simulink subsystem "Actuatormodel_R2019B"  (R2019b)
settings: Solver=VariableStepAuto  StartTime=0.0  StopTime=10.0  RelTol=1e-3
undefined symbols (not defined in the file): act, DiscIntNeverNeededParam
settings Model: Creator=dylaneijkelhof  LastModifiedBy=dylaneijkelhof

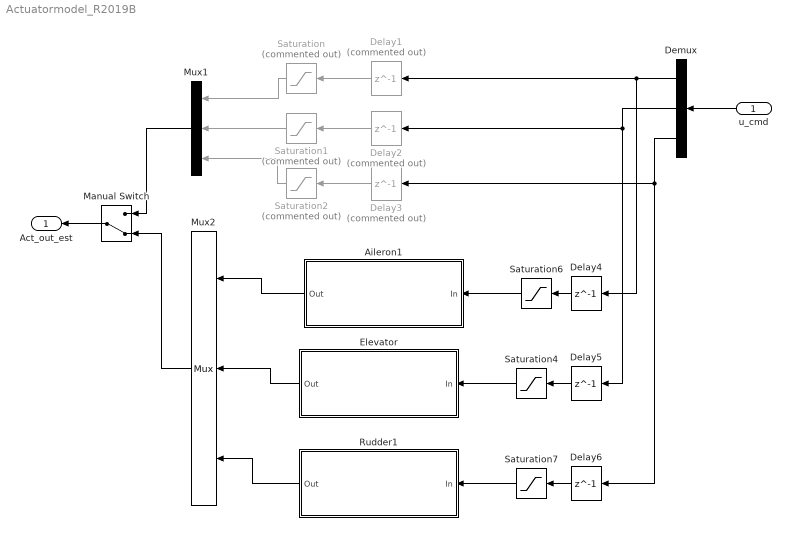
== system Actuatormodel_R2019B ==
  u_cmd : Inport
  Aileron1 : Subsystem  mask(Rate and Position Limited Servo){freq=act.aileron.w0/(2*pi), RL=act.aileron.rl, POS_hi=act.aileron.max_deflection, POS_lo=act.aileron.min_deflection, Bias=act.aileron.bias}
      mask prompts: freq "Bandwidth, Hz"; RL "Rate Limit:"; POS_hi "Position Limit High:"; POS_lo "Position Limit Low:"; Bias "Bias Value:"
      mask help:
      | First order transfer function: w/(s+w), with rate and position limits
      | and output bias level.
      mask Display:
      | text(.48,.55,sprintf('%3.1f Hz\nBW',freq),'horizontalAlignment','center');
      | 
      | text(0.18,0.45,sprintf('|d/dt|\n<%0.1f',RL),'horizontalAlignment','center');
      | 
      | text(0.88,0.85,num2str(POS_hi),'horizontalAlignment', 'center');
      | text(0.88,0.2,num2str(POS_lo),'horizontalAlignment', 'center');
      | text(0.73,0.5,'P\nL');
      | 
      | 
      | plot([0.83 0.87 0.93 0.97],[0.4 0.4 0.6 0.6]);
      | plot([0.81 0.99],[0.5 0.5]);
      | plot([0.9 0.9],[0.3 0.7]);
      | plot([0.81 0.99 0.99 0.81 0.81],[0.3 0.3 0.7 0.7 0.3]);
  Delay1 : Delay  Commented=on  DelayLength=1  InitialCondition=0
  Delay2 : Delay  Commented=on  DelayLength=1  InitialCondition=0
  Delay3 : Delay  Commented=on  DelayLength=1  InitialCondition=0
  Delay4 : Delay  DelayLength=1  InitialCondition=0
  Delay5 : Delay  DelayLength=1  InitialCondition=0
  Delay6 : Delay  DelayLength=1  InitialCondition=0
  Demux : Demux  Outputs=3
  Elevator : Subsystem  mask(Rate and Position Limited Servo){freq=act.elevator.w0/(2*pi), RL=act.elevator.rl, POS_hi=act.elevator.max_deflection, POS_lo=act.elevator.min_deflection, Bias=act.elevator.bias}
      mask prompts: freq "Bandwidth, Hz"; RL "Rate Limit:"; POS_hi "Position Limit High:"; POS_lo "Position Limit Low:"; Bias "Bias Value:"
      mask help:
      | First order transfer function: w/(s+w), with rate and position limits
      | and output bias level.
      mask Display:
      | text(.48,.55,sprintf('%3.1f Hz\nBW',freq),'horizontalAlignment','center');
      | 
      | text(0.18,0.45,sprintf('|d/dt|\n<%0.1f',RL),'horizontalAlignment','center');
      | 
      | text(0.88,0.85,num2str(POS_hi),'horizontalAlignment', 'center');
      | text(0.88,0.2,num2str(POS_lo),'horizontalAlignment', 'center');
      | text(0.73,0.5,'P\nL');
      | 
      | 
      | plot([0.83 0.87 0.93 0.97],[0.4 0.4 0.6 0.6]);
      | plot([0.81 0.99],[0.5 0.5]);
      | plot([0.9 0.9],[0.3 0.7]);
      | plot([0.81 0.99 0.99 0.81 0.81],[0.3 0.3 0.7 0.7 0.3]);
  Manual Switch : ManualSwitch  CurrentSetting=0
  Mux1 : Mux  Inputs=3
  Mux2 : Mux  Inputs=3
  Rudder1 : Subsystem  mask(Rate and Position Limited Servo){freq=act.rudder.w0/(2*pi), RL=act.rudder.rl, POS_hi=act.rudder.max_deflection, POS_lo=act.rudder.min_deflection, Bias=act.rudder.bias}
      mask prompts: freq "Bandwidth, Hz"; RL "Rate Limit:"; POS_hi "Position Limit High:"; POS_lo "Position Limit Low:"; Bias "Bias Value:"
      mask help:
      | First order transfer function: w/(s+w), with rate and position limits
      | and output bias level.
      mask Display:
      | text(.48,.55,sprintf('%3.1f Hz\nBW',freq),'horizontalAlignment','center');
      | 
      | text(0.18,0.45,sprintf('|d/dt|\n<%0.1f',RL),'horizontalAlignment','center');
      | 
      | text(0.88,0.85,num2str(POS_hi),'horizontalAlignment', 'center');
      | text(0.88,0.2,num2str(POS_lo),'horizontalAlignment', 'center');
      | text(0.73,0.5,'P\nL');
      | 
      | 
      | plot([0.83 0.87 0.93 0.97],[0.4 0.4 0.6 0.6]);
      | plot([0.81 0.99],[0.5 0.5]);
      | plot([0.9 0.9],[0.3 0.7]);
      | plot([0.81 0.99 0.99 0.81 0.81],[0.3 0.3 0.7 0.7 0.3]);
  Saturation : Saturate  Commented=on  UpperLimit=act.aileron.max_deflection  LowerLimit=act.aileron.min_deflection
  Saturation1 : Saturate  Commented=on  UpperLimit=act.elevator.max_deflection  LowerLimit=act.elevator.min_deflection
  Saturation2 : Saturate  Commented=on  UpperLimit=act.rudder.max_deflection  LowerLimit=act.rudder.min_deflection
  Saturation4 : Saturate  UpperLimit=act.elevator.max_deflection  LowerLimit=act.elevator.min_deflection
  Saturation6 : Saturate  UpperLimit=act.aileron.max_deflection  LowerLimit=act.aileron.min_deflection
  Saturation7 : Saturate  UpperLimit=act.rudder.max_deflection  LowerLimit=act.rudder.min_deflection
  Act_out_est : Outport  VectorParamsAs1DForOutWhenUnconnected=off
  wires:
  Demux/3 -> Delay3/1, Delay6/1
  Aileron1/1(Out) -> Mux2/1
  u_cmd/1 -> Demux/1
  Saturation2/1 -> Mux1/3
  Saturation4/1 -> Elevator/1(In)
  Delay2/1 -> Saturation1/1
  Delay6/1 -> Saturation7/1
  Demux/1 -> Delay4/1, Delay1/1
  Mux1/1 -> Manual Switch/1
  Demux/2 -> Delay2/1, Delay5/1
  Delay5/1 -> Saturation4/1
  Elevator/1(Out) -> Mux2/2
  Rudder1/1(Out) -> Mux2/3
  Saturation7/1 -> Rudder1/1(In)
  Saturation/1 -> Mux1/1
  Saturation6/1 -> Aileron1/1(In)
  Manual Switch/1 -> Act_out_est/1
  Delay1/1 -> Saturation/1
  Delay4/1 -> Saturation6/1
  Saturation1/1 -> Mux1/2
  Mux2/1 -> Manual Switch/2
  Delay3/1 -> Saturation2/1

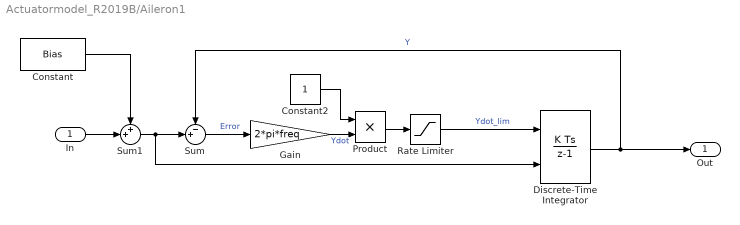
== system Actuatormodel_R2019B/Aileron1 ==
  In : Inport
  Constant : Constant  Value=Bias
  Constant2 : Constant
  Discrete-Time Integrator : DiscreteIntegrator  InitialConditionSource=external  SampleTime=-1  LimitOutput=on  UpperSaturationLimit=POS_hi  LowerSaturationLimit=POS_lo  ICPrevOutput=DiscIntNeverNeededParam  ICPrevScaledInput=DiscIntNeverNeededParam
  Gain : Gain  Gain=2*pi*freq  SaturateOnIntegerOverflow=on  OutDataTypeStr=Inherit: Same as input  ParamDataTypeStr=Inherit: Same as input
  Product : Product
  Rate Limiter : Saturate  UpperLimit=RL  LowerLimit=-RL
  Sum : Sum  Inputs=-+|  SaturateOnIntegerOverflow=on  InputSameDT=on  OutDataTypeStr=Inherit: Same as first input
  Sum1 : Sum  Inputs=++|  SaturateOnIntegerOverflow=on  InputSameDT=on  OutDataTypeStr=Inherit: Same as first input
  Out : Outport  PortDimensions=1  VectorParamsAs1DForOutWhenUnconnected=off
  wires:
  Product/1 -> Rate Limiter/1
  Sum1/1 -> Discrete-Time Integrator/2, Sum/2
  In/1 -> Sum1/2
  Rate Limiter/1 -> Discrete-Time Integrator/1  "Ydot_lim"
  Discrete-Time Integrator/1 -> Out/1, Sum/1  "Y"
  Sum/1 -> Gain/1  "Error"
  Gain/1 -> Product/2  "Ydot"
  Constant/1 -> Sum1/1
  Constant2/1 -> Product/1

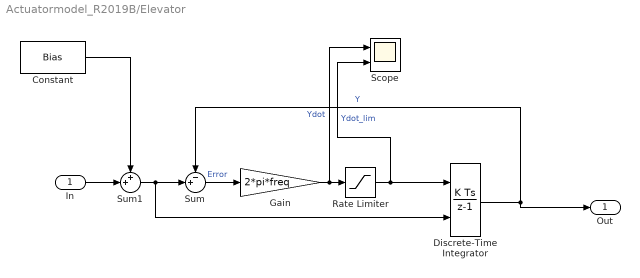
== system Actuatormodel_R2019B/Elevator ==
  In : Inport
  Constant : Constant  Value=Bias
  Discrete-Time Integrator : DiscreteIntegrator  InitialConditionSource=external  SampleTime=-1  LimitOutput=on  UpperSaturationLimit=POS_hi  LowerSaturationLimit=POS_lo  ICPrevOutput=DiscIntNeverNeededParam  ICPrevScaledInput=DiscIntNeverNeededParam
  Gain : Gain  Gain=2*pi*freq  SaturateOnIntegerOverflow=on  OutDataTypeStr=Inherit: Same as input  ParamDataTypeStr=Inherit: Same as input
  Rate Limiter : Saturate  UpperLimit=RL  LowerLimit=-RL
  Scope : Scope  NumInputPorts=2
  Sum : Sum  Inputs=-+|  SaturateOnIntegerOverflow=on  InputSameDT=on  OutDataTypeStr=Inherit: Same as first input
  Sum1 : Sum  Inputs=++|  SaturateOnIntegerOverflow=on  InputSameDT=on  OutDataTypeStr=Inherit: Same as first input
  Out : Outport  PortDimensions=1  VectorParamsAs1DForOutWhenUnconnected=off
  wires:
  Constant/1 -> Sum1/1
  Gain/1 -> Rate Limiter/1, Scope/1  "Ydot"
  Sum/1 -> Gain/1  "Error"
  Discrete-Time Integrator/1 -> Sum/1, Out/1  "Y"
  Rate Limiter/1 -> Discrete-Time Integrator/1, Scope/2  "Ydot_lim"
  In/1 -> Sum1/2
  Sum1/1 -> Sum/2, Discrete-Time Integrator/2

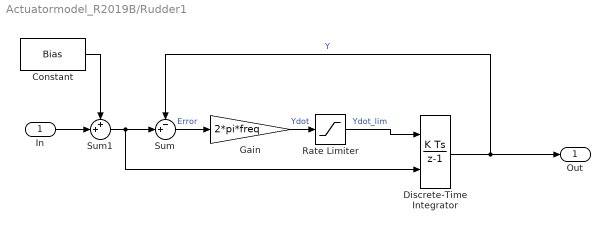
== system Actuatormodel_R2019B/Rudder1 ==
  In : Inport
  Constant : Constant  Value=Bias
  Discrete-Time Integrator : DiscreteIntegrator  InitialConditionSource=external  SampleTime=-1  LimitOutput=on  UpperSaturationLimit=POS_hi  LowerSaturationLimit=POS_lo  ICPrevOutput=DiscIntNeverNeededParam  ICPrevScaledInput=DiscIntNeverNeededParam
  Gain : Gain  Gain=2*pi*freq  SaturateOnIntegerOverflow=on  OutDataTypeStr=Inherit: Same as input  ParamDataTypeStr=Inherit: Same as input
  Rate Limiter : Saturate  UpperLimit=RL  LowerLimit=-RL
  Sum : Sum  Inputs=-+|  SaturateOnIntegerOverflow=on  InputSameDT=on  OutDataTypeStr=Inherit: Same as first input
  Sum1 : Sum  Inputs=++|  SaturateOnIntegerOverflow=on  InputSameDT=on  OutDataTypeStr=Inherit: Same as first input
  Out : Outport  PortDimensions=1  VectorParamsAs1DForOutWhenUnconnected=off
  wires:
  Gain/1 -> Rate Limiter/1  "Ydot"
  Sum/1 -> Gain/1  "Error"
  Discrete-Time Integrator/1 -> Sum/1, Out/1  "Y"
  Rate Limiter/1 -> Discrete-Time Integrator/1  "Ydot_lim"
  In/1 -> Sum1/2
  Sum1/1 -> Sum/2, Discrete-Time Integrator/2
  Constant/1 -> Sum1/1
